simulink model "IntelligentBinPicking"  (R2023a)
settings: Solver=FixedStepAuto  StartTime=0.0  StopTime=100  FixedStep=0.1  RelTol=1e-3
PreLoadFcn:
  | initializeParametersForBinPickingSimulationSL;
model workspace (MAT data in the model file):
  SL_ROS_VariableLengthArrays_MaxSizes.CommonInfo.ArrayTruncateAction = 'EmitWarning'
  SL_ROS_VariableLengthArrays_MaxSizes.MsgTypeMap = containers.Map
  SL_ROS_VariableLengthArrays_MaxSizes.MsgTypeMap.serialization.keys = {'sensor_msgs/Image', 'sensor_msgs/PointCloud2'}
  SL_ROS_VariableLengthArrays_MaxSizes.MsgTypeMap.serialization.values{1}(1).PropertyName = 'Data'
  SL_ROS_VariableLengthArrays_MaxSizes.MsgTypeMap.serialization.values{1}(1).DataType = 'uint8'
  SL_ROS_VariableLengthArrays_MaxSizes.MsgTypeMap.serialization.values{1}(1).MaxLength = 921600
  SL_ROS_VariableLengthArrays_MaxSizes.MsgTypeMap.serialization.values{1}(2).PropertyName = 'Encoding'
  SL_ROS_VariableLengthArrays_MaxSizes.MsgTypeMap.serialization.values{1}(2).DataType = 'uint8'
  SL_ROS_VariableLengthArrays_MaxSizes.MsgTypeMap.serialization.values{1}(2).MaxLength = 128
  SL_ROS_VariableLengthArrays_MaxSizes.MsgTypeMap.serialization.values{2}(1).PropertyName = 'Data'
  SL_ROS_VariableLengthArrays_MaxSizes.MsgTypeMap.serialization.values{2}(1).DataType = 'uint8'
  SL_ROS_VariableLengthArrays_MaxSizes.MsgTypeMap.serialization.values{2}(1).MaxLength = 9830400
  SL_ROS_VariableLengthArrays_MaxSizes.MsgTypeMap.serialization.values{2}(2).PropertyName = 'Fields'
  SL_ROS_VariableLengthArrays_MaxSizes.MsgTypeMap.serialization.values{2}(2).DataType = 'sensor_msgs/PointField'
  SL_ROS_VariableLengthArrays_MaxSizes.MsgTypeMap.serialization.values{2}(2).MaxLength = 16
  SL_ROS_VariableLengthArrays_MaxSizes.MsgTypeMap.serialization.uniformity = 0
  SL_ROS_VariableLengthArrays_MaxSizes.MsgTypeMap.serialization.keyType = 'char'
  SL_ROS_VariableLengthArrays_MaxSizes.MsgTypeMap.serialization.valueType = 'any'
undefined symbols (not defined in the file): binCenterPosition, Enable, enumCmd, homePosition, IsAccValid, IsMoving, IsPosValid, isSingleDetection, IsValid, IsVelValid, JointAcc, JointCurrent, JointPos, JointTrajectory, JointVel, maxVisionObjects, Mode, motionPlannerCmdInitValue, motionPlannerResponseInitValue, NumObjects, NumPoints, objectDetectorResponseInitValue, Objects, ObjectTypesID, PickAllOrder, pickAllOrder, PickAndPlaceModes, PickSelectedObjectID, posTargetError, RequestID, Reset, RGBCameraTransform, robotCommandInitValue, robotFeedbackInitValue, Status, targetEnv, TaskPlannerSampleTime, Time, TooltipTransform
libraries: robotlib x10, robotmaniplib x3, visionanalysis x2, robotcorelib x1, visiontextngfix x1, visionsinks x1
(part 1 of 2)
settings Model: Creator=gjohn  LastModifiedBy=amathamk
settings DebuggingCC: SubsystemReferenceDiagnosticForUnitTest=warning

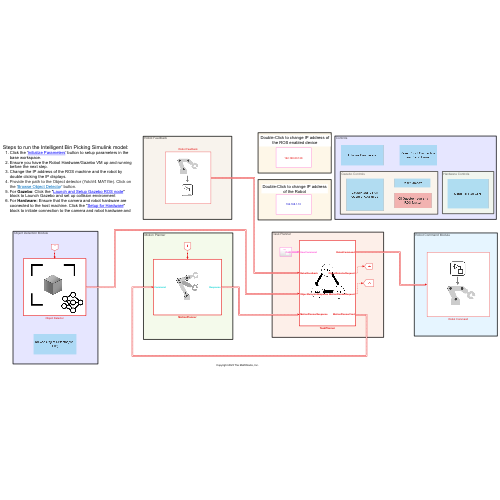
[thumbnail: Simulink's stored preview of the top-level diagram]
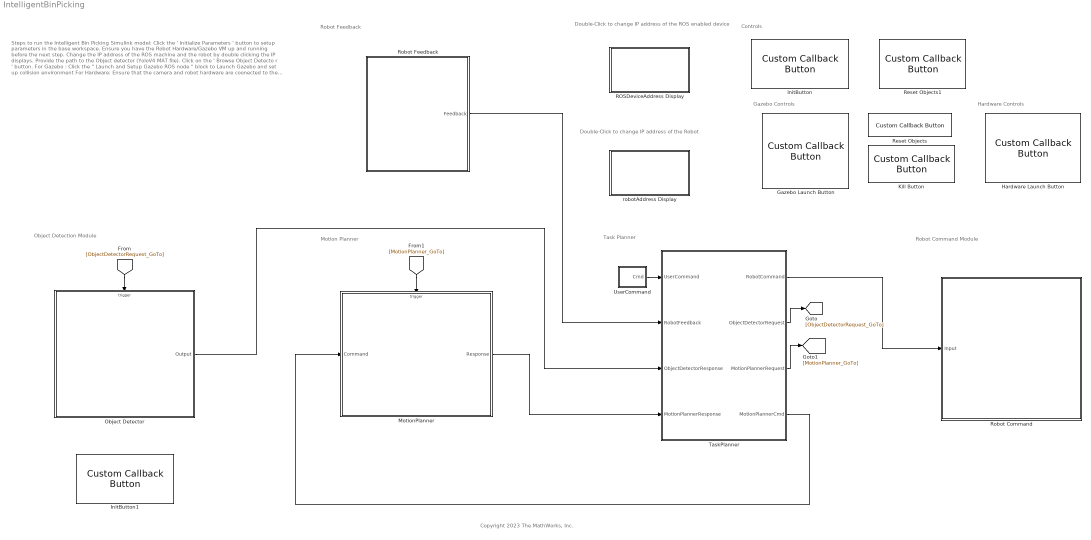
== system IntelligentBinPicking ==
  note: Double-Click to change IP address of the ROS enabled device
  note: Gazebo Controls
  note: Steps to run the Intelligent Bin Picking Simulink model:
      | Click the ' Initialize Parameters ' button to setup parameters in the base workspace.
      | Ensure you have the Robot Hardware/Gazebo VM up and running before the next step.
      | Change the IP address of the ROS machine and the robot by double clicking the IP displays.
      | Provide the path to the Object detector (YoloV4 MAT file). Click on the ' Browse Object Detecto r ' button.
      | For Gazebo : Click the " Launch and Setup Gazebo ROS node " block to Launch Gazebo and set up collision environment
      | For Hardware: Ensure that the camera and robot hardware are coonected to the host machine. Click the " Setup for Hardware " block to initiate connection to the camera and robot hardware and call rosinit.
  note: Task Planner
  note: Motion Planner
  note: Robot Command Module
  note: Robot Feedback
  note: Object Detection Module
  note: Controls
  note: Copyright 2023 The MathWorks, Inc.
  note: Hardware Controls
  note: Double-Click to change IP address of the Robot
  Gazebo Launch Button : CustomCallbackButton  Configuration="{\"components\":[{\"name\":\"BackgroundImageComponent\",\"settings\":{\"image\":{\"size\":[0,0],\"src\":\"default\",\"srcOrientation\":\"Right\"},\"position\":[0,0,1,1]}},{\"name\":\"ButtonStateComponent\",\"settings\":{\"buttonType\":\"momentary\",\"clickFcn\":\"LaunchGazeboAndSetupCollisionEnv;\\ndisp(\\\"Gazebo launched and scene setup\\\")\\n\",\"onValue\":1,\"position\":[0,0,1,1],\"pressDelay\":\"500\",\"pressFcn\":\"\",\"repeatInterval\":\"0\",\"states\":[{\"horizontalAlignment\":\"center\",\"image\":{\"position\":[0,0,1,1],\"size\":[1,1],\"src\":\"default\",\"srcOrientation\":\"Right\"},\"label\":{\"color\":[0.01176470588,0.01176470588,0.01176470588,1],\"icon\":{\"size\":[0,0],\"src\":\"default\",\"srcOrientation\":\"Right\"},\"iconPlacement\":\"left\",\"opacity\":1,\"show\":true,\"text\":{\"content\":\"Launch and Setup Gazebo ROS node\",\"font\":\"Helvetica\",\"fontSize\":9.600000000000001}},\"labelOffset\":[0,0],\"verticalAlignment\":\"middle\"},{\"horizontalAlignment\":\"center\",\"image\":{\"position\":[0,0,1,1],\"size\":[1,1],\"src\":\"default\",\"srcOrientation\":\"Right\"},\"label\":{\"color\":[0.01176470588,0.01176470588,0.01176470588,1],\"icon\":{\"size\":[0,0],\"src\":\"default\",\"srcOrientation\":\"Right\"},\"iconPlacement\":\"left\",\"opacity\":1,\"show\":true,\"text\":{\"content\":\"Launch and Setup Gazebo ROS node\",\"font\":\"Helvetica\",\"fontSize\":9.600000000000001}},\"labelOffset\":[0,0],\"verticalAlignment\":\"middle\"},{\"horizontalAlignment\":\"center\",\"image\":{\"position\":[0,0,1,1],\"size\":[1,1],\"src\":\"default\",\"srcOrientation\":\"Right\"},\"label\":{\"color\":[0.01176470588,0.01176470588,0.01176470588,1],\"icon\":{\"size\":[0,0],\"src\":\"default\",\"srcOrientation\":\"Right\"},\"iconPlacement\":\"left\",\"opacity\":1,\"show\":true,\"text\":{\"content\":\"Launch and Setup Gazebo ROS node\",\"font\":\"Helvetica\",\"fontSize\":9.600000000000001}},\"labelOffset\":[0,0],\"verticalAlignment\":\"middle\"},{\"horizontalAlignment\":\"center\",\"image\":{\"position\":[0,0,1,1],\"size\":[1,1],\"src\":\"default\",\"srcOrientation\":\"Right\"},\"label\":{\"color\":[0.01176470588,0.01176470588,0.01176470588,1],\"icon\":{\"size\":[0,0],\"src\":\"default\",\"srcOrientation\":\"Right\"},\"iconPlacement\":\"left\",\"opacity\":1,\"show\":true,\"text\":{\"content\":\"Launch and Setup Gazebo ROS node\",\"font\":\"Helvetica\",\"fontSize\":9.600000000000001}},\"labelOffset\":[0,0],\"verticalAlignment\":\"middle\"}]}},{\"name\":\"ForegroundImageComponent\",\"settings\":{\"image\":{\"size\":[0,0],\"src\":\"default\",\"srcOrientation\":\"Right\"},\"isForeground\":1,\"position\":[0,0,1,1]}}],\"settings\":{\"BindingType\":\"standalone\",\"backgroundColor\":[244,244,244,1],\"backgroundOffset\":0,\"backgroundOpacity\":1,\"fixedAspectRatio\":\"off\",\"foregroundColor\":[0.01176470588,0.01176470588,0.01176470588,1],\"migratedFromLegacy\":true,\"useBackgroundColor\":true,\"variant\":\"callback\",\"version\":\"R2023a\"},\"type\":\"Button\"}"  CustomBackgroundColor="{\"color\":[0.6196078431372549,0.8392156862745098,0.9490196078431372],\"show\":true}"
  Hardware Launch Button : CustomCallbackButton  Configuration="{\"components\":[{\"name\":\"BackgroundImageComponent\",\"settings\":{\"image\":{\"size\":[0,0],\"src\":\"default\",\"srcOrientation\":\"Right\"},\"position\":[0,0,1,1]}},{\"name\":\"ButtonStateComponent\",\"settings\":{\"buttonType\":\"momentary\",\"clickFcn\":\"getGripperType;\\n\\nConnectToRobotROS;\\n\\ndisp(\\\"Setup complete for Robot hardware\\\")\\n\",\"onValue\":1,\"position\":[0,0,1,1],\"pressDelay\":\"500\",\"pressFcn\":\"\",\"repeatInterval\":\"0\",\"states\":[{\"horizontalAlignment\":\"center\",\"image\":{\"position\":[0,0,1,1],\"size\":[1,1],\"src\":\"default\",\"srcOrientation\":\"Right\"},\"label\":{\"color\":[0.011764705882352941,0.011764705882352941,0.011764705882352941],\"icon\":{\"size\":[0,0],\"src\":\"default\",\"srcOrientation\":\"Right\"},\"iconPlacement\":\"left\",\"opacity\":1,\"show\":true,\"text\":{\"content\":\"Setup for Hardware\",\"font\":\"Helvetica\",\"fontSize\":11.709468000000001}},\"labelOffset\":[0,0],\"verticalAlignment\":\"middle\"},{\"horizontalAlignment\":\"center\",\"image\":{\"position\":[0,0,1,1],\"size\":[1,1],\"src\":\"default\",\"srcOrientation\":\"Right\"},\"label\":{\"color\":[0.011764705882352941,0.011764705882352941,0.011764705882352941],\"icon\":{\"size\":[0,0],\"src\":\"default\",\"srcOrientation\":\"Right\"},\"iconPlacement\":\"left\",\"opacity\":1,\"show\":true,\"text\":{\"content\":\"Setup for Hardware\",\"font\":\"Helvetica\",\"fontSize\":11.709468000000001}},\"labelOffset\":[0,0],\"verticalAlignment\":\"middle\"},{\"horizontalAlignment\":\"center\",\"image\":{\"position\":[0,0,1,1],\"size\":[1,1],\"src\":\"default\",\"srcOrientation\":\"Right\"},\"label\":{\"color\":[0.011764705882352941,0.011764705882352941,0.011764705882352941],\"icon\":{\"size\":[0,0],\"src\":\"default\",\"srcOrientation\":\"Right\"},\"iconPlacement\":\"left\",\"opacity\":1,\"show\":true,\"text\":{\"content\":\"Setup for Hardware\",\"font\":\"Helvetica\",\"fontSize\":11.709468000000001}},\"labelOffset\":[0,0],\"verticalAlignment\":\"middle\"},{\"horizontalAlignment\":\"center\",\"image\":{\"position\":[0,0,1,1],\"size\":[1,1],\"src\":\"default\",\"srcOrientation\":\"Right\"},\"label\":{\"color\":[0.011764705882352941,0.011764705882352941,0.011764705882352941],\"icon\":{\"size\":[0,0],\"src\":\"default\",\"srcOrientation\":\"Right\"},\"iconPlacement\":\"left\",\"opacity\":1,\"show\":true,\"text\":{\"content\":\"Setup for Hardware\",\"font\":\"Helvetica\",\"fontSize\":11.709468000000001}},\"labelOffset\":[0,0],\"verticalAlignment\":\"middle\"}]}},{\"name\":\"ForegroundImageComponent\",\"settings\":{\"image\":{\"size\":[0,0],\"src\":\"default\",\"srcOrientation\":\"Right\"},\"isForeground\":1,\"position\":[0,0,1,1]}}],\"settings\":{\"BindingType\":\"standalone\",\"backgroundColor\":[244,244,244,1],\"backgroundOffset\":0,\"backgroundOpacity\":1,\"fixedAspectRatio\":\"off\",\"foregroundColor\":[0.01176470588,0.01176470588,0.01176470588,1],\"migratedFromLegacy\":true,\"useBackgroundColor\":true,\"variant\":\"callback\",\"version\":\"R2023a\"},\"type\":\"Button\"}"  CustomBackgroundColor="{\"color\":[0.6196078431372549,0.8392156862745098,0.9490196078431372],\"show\":true}"
  InitButton : CustomCallbackButton  Configuration="{\"components\":[{\"name\":\"BackgroundImageComponent\",\"settings\":{\"image\":{\"size\":[0,0],\"src\":\"default\",\"srcOrientation\":\"Right\"},\"position\":[0,0,1,1]}},{\"name\":\"ButtonStateComponent\",\"settings\":{\"buttonType\":\"momentary\",\"clickFcn\":\"%%\\ninitializeParametersForBinPickingSimulationSL;\\ndisp('Parameters Initialized')\",\"onValue\":1,\"position\":[0,0,1,1],\"pressDelay\":\"500\",\"pressFcn\":\"\",\"repeatInterval\":\"0\",\"states\":[{\"horizontalAlignment\":\"center\",\"image\":{\"position\":[0,0,1,1],\"size\":[1,1],\"src\":\"default\",\"srcOrientation\":\"Right\"},\"label\":{\"color\":[0,0,0],\"icon\":{\"size\":[0,0],\"src\":\"default\",\"srcOrientation\":\"Right\"},\"iconPlacement\":\"left\",\"opacity\":1,\"show\":true,\"text\":{\"content\":\"Initialize Parameters\",\"font\":\"Helvetica\",\"fontSize\":11.709468000000001}},\"labelOffset\":[0,0],\"verticalAlignment\":\"middle\"},{\"horizontalAlignment\":\"center\",\"image\":{\"position\":[0,0,1,1],\"size\":[1,1],\"src\":\"default\",\"srcOrientation\":\"Right\"},\"label\":{\"color\":[0.01176470588,0.01176470588,0.01176470588,1],\"icon\":{\"size\":[0,0],\"src\":\"default\",\"srcOrientation\":\"Right\"},\"iconPlacement\":\"left\",\"opacity\":1,\"show\":true,\"text\":{\"content\":\"Initialize Parameters\",\"font\":\"Helvetica\",\"fontSize\":11.709468000000001}},\"labelOffset\":[0,0],\"verticalAlignment\":\"middle\"},{\"horizontalAlignment\":\"center\",\"image\":{\"position\":[0,0,1,1],\"size\":[1,1],\"src\":\"default\",\"srcOrientation\":\"Right\"},\"label\":{\"color\":[0.01176470588,0.01176470588,0.01176470588,1],\"icon\":{\"size\":[0,0],\"src\":\"default\",\"srcOrientation\":\"Right\"},\"iconPlacement\":\"left\",\"opacity\":1,\"show\":true,\"text\":{\"content\":\"Initialize Parameters\",\"font\":\"Helvetica\",\"fontSize\":11.709468000000001}},\"labelOffset\":[0,0],\"verticalAlignment\":\"middle\"},{\"horizontalAlignment\":\"center\",\"image\":{\"position\":[0,0,1,1],\"size\":[1,1],\"src\":\"default\",\"srcOrientation\":\"Right\"},\"label\":{\"color\":[0.01176470588,0.01176470588,0.01176470588,1],\"icon\":{\"size\":[0,0],\"src\":\"default\",\"srcOrientation\":\"Right\"},\"iconPlacement\":\"left\",\"opacity\":1,\"show\":true,\"text\":{\"content\":\"Initialize Parameters\",\"font\":\"Helvetica\",\"fontSize\":11.709468000000001}},\"labelOffset\":[0,0],\"verticalAlignment\":\"middle\"}]}},{\"name\":\"ForegroundImageComponent\",\"settings\":{\"image\":{\"size\":[0,0],\"src\":\"default\",\"srcOrientation\":\"Right\"},\"isForeground\":1,\"position\":[0,0,1,1]}}],\"settings\":{\"BindingType\":\"standalone\",\"backgroundColor\":[244,244,244,1],\"backgroundOffset\":0,\"backgroundOpacity\":1,\"fixedAspectRatio\":\"off\",\"foregroundColor\":[0.01176470588,0.01176470588,0.01176470588,1],\"migratedFromLegacy\":true,\"useBackgroundColor\":true,\"variant\":\"callback\",\"version\":\"R2023a\"},\"type\":\"Button\"}"  CustomBackgroundColor="{\"color\":[0.6196078431372549,0.8392156862745098,0.9490196078431372],\"show\":true}"
  InitButton1 : CustomCallbackButton  Configuration="{\"components\":[{\"name\":\"BackgroundImageComponent\",\"settings\":{\"image\":{\"size\":[0,0],\"src\":\"default\",\"srcOrientation\":\"Right\"},\"position\":[0,0,1,1]}},{\"name\":\"ButtonStateComponent\",\"settings\":{\"buttonType\":\"momentary\",\"clickFcn\":\"selectDetectorMATFile\",\"onValue\":1,\"position\":[0,0,1,1],\"pressDelay\":\"500\",\"pressFcn\":\"\",\"repeatInterval\":\"0\",\"states\":[{\"horizontalAlignment\":\"center\",\"image\":{\"position\":[0,0,1,1],\"size\":[1,1],\"src\":\"default\",\"srcOrientation\":\"Right\"},\"label\":{\"color\":[0,0,0],\"icon\":{\"size\":[0,0],\"src\":\"default\",\"srcOrientation\":\"Right\"},\"iconPlacement\":\"left\",\"opacity\":1,\"show\":true,\"text\":{\"content\":\"Browse Object Detector(MAT File)\",\"font\":\"Helvetica\",\"fontSize\":10.608108000000001}},\"labelOffset\":[0,0],\"verticalAlignment\":\"middle\"},{\"horizontalAlignment\":\"center\",\"image\":{\"position\":[0,0,1,1],\"size\":[1,1],\"src\":\"default\",\"srcOrientation\":\"Right\"},\"label\":{\"color\":[0.01176470588,0.01176470588,0.01176470588,1],\"icon\":{\"size\":[0,0],\"src\":\"default\",\"srcOrientation\":\"Right\"},\"iconPlacement\":\"left\",\"opacity\":1,\"show\":true,\"text\":{\"content\":\"Browse Object Detector(MAT File)\",\"font\":\"Helvetica\",\"fontSize\":10.608108000000001}},\"labelOffset\":[0,0],\"verticalAlignment\":\"middle\"},{\"horizontalAlignment\":\"center\",\"image\":{\"position\":[0,0,1,1],\"size\":[1,1],\"src\":\"default\",\"srcOrientation\":\"Right\"},\"label\":{\"color\":[0.01176470588,0.01176470588,0.01176470588,1],\"icon\":{\"size\":[0,0],\"src\":\"default\",\"srcOrientation\":\"Right\"},\"iconPlacement\":\"left\",\"opacity\":1,\"show\":true,\"text\":{\"content\":\"Browse Object Detector(MAT File)\",\"font\":\"Helvetica\",\"fontSize\":10.608108000000001}},\"labelOffset\":[0,0],\"verticalAlignment\":\"middle\"},{\"horizontalAlignment\":\"center\",\"image\":{\"position\":[0,0,1,1],\"size\":[1,1],\"src\":\"default\",\"srcOrientation\":\"Right\"},\"label\":{\"color\":[0.01176470588,0.01176470588,0.01176470588,1],\"icon\":{\"size\":[0,0],\"src\":\"default\",\"srcOrientation\":\"Right\"},\"iconPlacement\":\"left\",\"opacity\":1,\"show\":true,\"text\":{\"content\":\"Browse Object Detector(MAT File)\",\"font\":\"Helvetica\",\"fontSize\":10.608108000000001}},\"labelOffset\":[0,0],\"verticalAlignment\":\"middle\"}]}},{\"name\":\"ForegroundImageComponent\",\"settings\":{\"image\":{\"size\":[0,0],\"src\":\"default\",\"srcOrientation\":\"Right\"},\"isForeground\":1,\"position\":[0,0,1,1]}}],\"settings\":{\"BindingType\":\"standalone\",\"backgroundColor\":[244,244,244,1],\"backgroundOffset\":0,\"backgroundOpacity\":1,\"fixedAspectRatio\":\"off\",\"foregroundColor\":[0.01176470588,0.01176470588,0.01176470588,1],\"migratedFromLegacy\":true,\"useBackgroundColor\":true,\"variant\":\"callback\",\"version\":\"R2023a\"},\"type\":\"Button\"}"  CustomBackgroundColor="{\"color\":[0.6196078431372549,0.8392156862745098,0.9490196078431372],\"show\":true}"
  Kill Button : CustomCallbackButton  Configuration="{\"components\":[{\"name\":\"BackgroundImageComponent\",\"settings\":{\"image\":{\"size\":[0,0],\"src\":\"default\",\"srcOrientation\":\"Right\"},\"position\":[0,0,1,1]}},{\"name\":\"ButtonStateComponent\",\"settings\":{\"buttonType\":\"momentary\",\"clickFcn\":\"clear ur\\nurHandleClass.manageURNodeMap(ROSDeviceAddress,[],'remove')\\nif exist('device', 'var')\\n    system(device,'killall -9 rosmaster');\\nend\",\"onValue\":1,\"position\":[0,0,1,1],\"pressDelay\":\"500\",\"pressFcn\":\"\",\"repeatInterval\":\"0\",\"states\":[{\"horizontalAlignment\":\"center\",\"image\":{\"position\":[0,0,1,1],\"size\":[1,1],\"src\":\"default\",\"srcOrientation\":\"Right\"},\"label\":{\"color\":[0,0,0],\"icon\":{\"size\":[0,0],\"src\":\"default\",\"srcOrientation\":\"Right\"},\"iconPlacement\":\"left\",\"opacity\":1,\"show\":true,\"text\":{\"content\":\"Kill Gazebo node and ROS Master\",\"font\":\"Helvetica\",\"fontSize\":14.45202}},\"labelOffset\":[0,0],\"verticalAlignment\":\"middle\"},{\"horizontalAlignment\":\"center\",\"image\":{\"position\":[0,0,1,1],\"size\":[1,1],\"src\":\"default\",\"srcOrientation\":\"Right\"},\"label\":{\"color\":[0.01176470588,0.01176470588,0.01176470588,1],\"icon\":{\"size\":[0,0],\"src\":\"default\",\"srcOrientation\":\"Right\"},\"iconPlacement\":\"left\",\"opacity\":1,\"show\":true,\"text\":{\"content\":\"Kill Gazebo node and ROS Master\",\"font\":\"Helvetica\",\"fontSize\":14.45202}},\"labelOffset\":[0,0],\"verticalAlignment\":\"middle\"},{\"horizontalAlignment\":\"center\",\"image\":{\"position\":[0,0,1,1],\"size\":[1,1],\"src\":\"default\",\"srcOrientation\":\"Right\"},\"label\":{\"color\":[0.01176470588,0.01176470588,0.01176470588,1],\"icon\":{\"size\":[0,0],\"src\":\"default\",\"srcOrientation\":\"Right\"},\"iconPlacement\":\"left\",\"opacity\":1,\"show\":true,\"text\":{\"content\":\"Kill Gazebo node and ROS Master\",\"font\":\"Helvetica\",\"fontSize\":14.45202}},\"labelOffset\":[0,0],\"verticalAlignment\":\"middle\"},{\"horizontalAlignment\":\"center\",\"image\":{\"position\":[0,0,1,1],\"size\":[1,1],\"src\":\"default\",\"srcOrientation\":\"Right\"},\"label\":{\"color\":[0.01176470588,0.01176470588,0.01176470588,1],\"icon\":{\"size\":[0,0],\"src\":\"default\",\"srcOrientation\":\"Right\"},\"iconPlacement\":\"left\",\"opacity\":1,\"show\":true,\"text\":{\"content\":\"Kill Gazebo node and ROS Master\",\"font\":\"Helvetica\",\"fontSize\":14.45202}},\"labelOffset\":[0,0],\"verticalAlignment\":\"middle\"}]}},{\"name\":\"ForegroundImageComponent\",\"settings\":{\"image\":{\"size\":[0,0],\"src\":\"default\",\"srcOrientation\":\"Right\"},\"isForeground\":1,\"position\":[0,0,1,1]}}],\"settings\":{\"BindingType\":\"standalone\",\"backgroundColor\":[244,244,244,1],\"backgroundOffset\":0,\"backgroundOpacity\":1,\"fixedAspectRatio\":\"off\",\"foregroundColor\":[0.01176470588,0.01176470588,0.01176470588,1],\"migratedFromLegacy\":true,\"useBackgroundColor\":true,\"variant\":\"callback\",\"version\":\"R2023a\"},\"type\":\"Button\"}"  CustomBackgroundColor="{\"color\":[0.9411764705882353,0.6313725490196078,0.6313725490196078],\"show\":true}"
  MotionPlanner : Subsystem
      mask Display: image('$imagefile'); % Use "Edit Image" on toolstrip to change.
  Object Detector : Subsystem  TreatAsAtomicUnit=on
      mask Display: image('$imagefile'); % Use "Edit Image" on toolstrip to change.
  ROSDeviceAddress Display : Subsystem
      settings: OpenFcn=RequestIP;
      mask Display: color('red'); try ipad = evalin('base', 'ROSDeviceAddress'); catch ipad = '0.0.0.0'; end; disp(ipad)
  Reset Objects : CustomCallbackButton  Configuration="{\"components\":[{\"name\":\"BackgroundImageComponent\",\"settings\":{\"image\":{\"size\":[0,0],\"src\":\"default\",\"srcOrientation\":\"Right\"},\"position\":[0,0,1,1]}},{\"name\":\"ButtonStateComponent\",\"settings\":{\"buttonType\":\"momentary\",\"clickFcn\":\"ResetObjectsGazebo;\\ndisp(\\\"Object positions and collision environment reset\\\")\",\"onValue\":1,\"position\":[0,0,1,1],\"pressDelay\":\"500\",\"pressFcn\":\"\",\"repeatInterval\":\"0\",\"states\":[{\"horizontalAlignment\":\"center\",\"image\":{\"position\":[0,0,1,1],\"size\":[1,1],\"src\":\"default\",\"srcOrientation\":\"Right\"},\"label\":{\"color\":[0,0,0],\"icon\":{\"size\":[0,0],\"src\":\"default\",\"srcOrientation\":\"Right\"},\"iconPlacement\":\"left\",\"opacity\":1,\"show\":true,\"text\":{\"content\":\"Reset Objects\",\"font\":\"Helvetica\",\"fontSize\":15}},\"labelOffset\":[0,0],\"verticalAlignment\":\"middle\"},{\"horizontalAlignment\":\"center\",\"image\":{\"position\":[0,0,1,1],\"size\":[1,1],\"src\":\"default\",\"srcOrientation\":\"Right\"},\"label\":{\"color\":[0.01176470588,0.01176470588,0.01176470588,1],\"icon\":{\"size\":[0,0],\"src\":\"default\",\"srcOrientation\":\"Right\"},\"iconPlacement\":\"left\",\"opacity\":1,\"show\":true,\"text\":{\"content\":\"Reset Objects\",\"font\":\"Helvetica\",\"fontSize\":15}},\"labelOffset\":[0,0],\"verticalAlignment\":\"middle\"},{\"horizontalAlignment\":\"center\",\"image\":{\"position\":[0,0,1,1],\"size\":[1,1],\"src\":\"default\",\"srcOrientation\":\"Right\"},\"label\":{\"color\":[0.01176470588,0.01176470588,0.01176470588,1],\"icon\":{\"size\":[0,0],\"src\":\"default\",\"srcOrientation\":\"Right\"},\"iconPlacement\":\"left\",\"opacity\":1,\"show\":true,\"text\":{\"content\":\"Reset Objects\",\"font\":\"Helvetica\",\"fontSize\":15}},\"labelOffset\":[0,0],\"verticalAlignment\":\"middle\"},{\"horizontalAlignment\":\"center\",\"image\":{\"position\":[0,0,1,1],\"size\":[1,1],\"src\":\"default\",\"srcOrientation\":\"Right\"},\"label\":{\"color\":[0.01176470588,0.01176470588,0.01176470588,1],\"icon\":{\"size\":[0,0],\"src\":\"default\",\"srcOrientation\":\"Right\"},\"iconPlacement\":\"left\",\"opacity\":1,\"show\":true,\"text\":{\"content\":\"Reset Objects\",\"font\":\"Helvetica\",\"fontSize\":15}},\"labelOffset\":[0,0],\"verticalAlignment\":\"middle\"}]}},{\"name\":\"ForegroundImageComponent\",\"settings\":{\"image\":{\"size\":[0,0],\"src\":\"default\",\"srcOrientation\":\"Right\"},\"isForeground\":1,\"position\":[0,0,1,1]}}],\"settings\":{\"BindingType\":\"standalone\",\"backgroundColor\":[244,244,244,1],\"backgroundOffset\":0,\"backgroundOpacity\":1,\"fixedAspectRatio\":\"off\",\"foregroundColor\":[0.01176470588,0.01176470588,0.01176470588,1],\"migratedFromLegacy\":true,\"useBackgroundColor\":true,\"variant\":\"callback\",\"version\":\"R2023a\"},\"type\":\"Button\"}"  CustomBackgroundColor="{\"color\":[0.6196078431372549,0.8392156862745098,0.9490196078431372],\"show\":true}"
  Reset Objects1 : CustomCallbackButton  Configuration="{\"components\":[{\"name\":\"BackgroundImageComponent\",\"settings\":{\"image\":{\"size\":[0,0],\"src\":\"default\",\"srcOrientation\":\"Right\"},\"position\":[0,0,1,1]}},{\"name\":\"ButtonStateComponent\",\"settings\":{\"buttonType\":\"momentary\",\"clickFcn\":\"urHandleClass.manageURNodeMap(ROSDeviceAddress,[],'remove');\\nif exist('ur', 'var')\\n    clear ur\\nend\\nur = universalrobot(ROSDeviceAddress,'RigidBodyTree',ur5e);\\nsendJointConfigurationAndWait(ur,homePosition,'EndTime',2);\\npause(2);\\nclear ur\\ndisp(\\\"Robot connection reset\\\")\",\"onValue\":1,\"position\":[0,0,1,1],\"pressDelay\":\"500\",\"pressFcn\":\"\",\"repeatInterval\":\"0\",\"states\":[{\"horizontalAlignment\":\"center\",\"image\":{\"position\":[0,0,1,1],\"size\":[1,1],\"src\":\"default\",\"srcOrientation\":\"Right\"},\"label\":{\"color\":[0,0,0],\"icon\":{\"size\":[0,0],\"src\":\"default\",\"srcOrientation\":\"Right\"},\"iconPlacement\":\"left\",\"opacity\":1,\"show\":true,\"text\":{\"content\":\"Reset Robot Connection and Send Home\",\"font\":\"Helvetica\",\"fontSize\":14.45202}},\"labelOffset\":[0,0],\"verticalAlignment\":\"middle\"},{\"horizontalAlignment\":\"center\",\"image\":{\"position\":[0,0,1,1],\"size\":[1,1],\"src\":\"default\",\"srcOrientation\":\"Right\"},\"label\":{\"color\":[0.01176470588,0.01176470588,0.01176470588,1],\"icon\":{\"size\":[0,0],\"src\":\"default\",\"srcOrientation\":\"Right\"},\"iconPlacement\":\"left\",\"opacity\":1,\"show\":true,\"text\":{\"content\":\"Reset Robot Connection and Send Home\",\"font\":\"Helvetica\",\"fontSize\":14.45202}},\"labelOffset\":[0,0],\"verticalAlignment\":\"middle\"},{\"horizontalAlignment\":\"center\",\"image\":{\"position\":[0,0,1,1],\"size\":[1,1],\"src\":\"default\",\"srcOrientation\":\"Right\"},\"label\":{\"color\":[0.01176470588,0.01176470588,0.01176470588,1],\"icon\":{\"size\":[0,0],\"src\":\"default\",\"srcOrientation\":\"Right\"},\"iconPlacement\":\"left\",\"opacity\":1,\"show\":true,\"text\":{\"content\":\"Reset Robot Connection and Send Home\",\"font\":\"Helvetica\",\"fontSize\":14.45202}},\"labelOffset\":[0,0],\"verticalAlignment\":\"middle\"},{\"horizontalAlignment\":\"center\",\"image\":{\"position\":[0,0,1,1],\"size\":[1,1],\"src\":\"default\",\"srcOrientation\":\"Right\"},\"label\":{\"color\":[0.01176470588,0.01176470588,0.01176470588,1],\"icon\":{\"size\":[0,0],\"src\":\"default\",\"srcOrientation\":\"Right\"},\"iconPlacement\":\"left\",\"opacity\":1,\"show\":true,\"text\":{\"content\":\"Reset Robot Connection and Send Home\",\"font\":\"Helvetica\",\"fontSize\":14.45202}},\"labelOffset\":[0,0],\"verticalAlignment\":\"middle\"}]}},{\"name\":\"ForegroundImageComponent\",\"settings\":{\"image\":{\"size\":[0,0],\"src\":\"default\",\"srcOrientation\":\"Right\"},\"isForeground\":1,\"position\":[0,0,1,1]}}],\"settings\":{\"BindingType\":\"standalone\",\"backgroundColor\":[244,244,244,1],\"backgroundOffset\":0,\"backgroundOpacity\":1,\"fixedAspectRatio\":\"off\",\"foregroundColor\":[0.01176470588,0.01176470588,0.01176470588,1],\"migratedFromLegacy\":true,\"useBackgroundColor\":true,\"variant\":\"callback\",\"version\":\"R2023a\"},\"type\":\"Button\"}"  CustomBackgroundColor="{\"color\":[0.615686274509804,0.8392156862745098,0.9490196078431372],\"show\":true}"
  Robot Command : Subsystem
      mask Display: image('SLToRobotComm.png'); % Use "Edit Image" on toolstrip to change.
  Robot Feedback : Subsystem
      mask Display: image('$imagefile'); % Use "Edit Image" on toolstrip to change.
  TaskPlanner : Subsystem  TreatAsAtomicUnit=on  SystemSampleTime=TaskPlannerSampleTime
      mask Display: image('$imagefile'); % Use "Edit Image" on toolstrip to change.
  UserCommand : Subsystem
  robotAddress Display : Subsystem
      settings: OpenFcn=RequestRobotIP;
      mask Display: color('blue'); try ipad = evalin('base', 'robotAddress'); catch ipad = '192.162.1.10'; end; disp(ipad)
  wires:
  UserCommand/1(Cmd) -> TaskPlanner/1(UserCommand)
  TaskPlanner/2(ObjectDetectorRequest) -> [ObjectDetectorRequest_GoTo]
  [ObjectDetectorRequest_GoTo] -> Object Detector/Trigger
  TaskPlanner/3(MotionPlannerRequest) -> [MotionPlanner_GoTo]
  [MotionPlanner_GoTo] -> MotionPlanner/Trigger
  TaskPlanner/1(RobotCommand) -> Robot Command/1(Input)
  TaskPlanner/4(MotionPlannerCmd) -> MotionPlanner/1(Command)
  MotionPlanner/1(Response) -> TaskPlanner/4(MotionPlannerResponse)
  Object Detector/1(Output) -> TaskPlanner/3(ObjectDetectorResponse)
  Robot Feedback/1(Feedback) -> TaskPlanner/2(RobotFeedback)

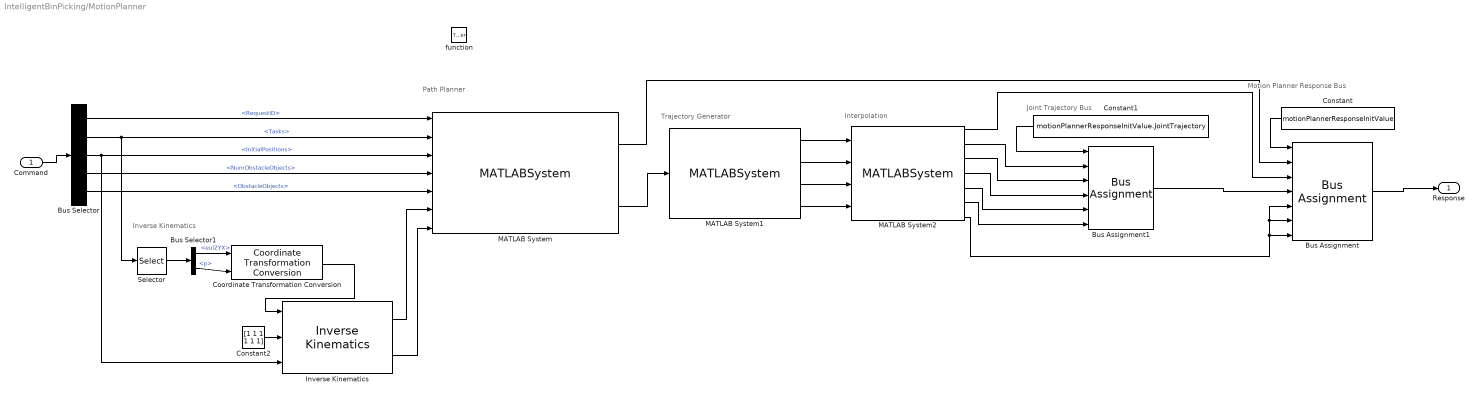
== system IntelligentBinPicking/MotionPlanner ==
  note: Interpolation
  note: Trajectory Generator
  note: Path Planner
  note: Inverse Kinematics
  note: Joint Trajectory Bus
  note: Motion Planner Response Bus
  Command : Inport  OutDataTypeStr=Bus: BUS_motion_planner_cmd
  function : TriggerPort  TriggerType=function-call  VariantControl=Variant  PortDimensions=1
  Bus Assignment : BusAssignment  AssignedSignals=RequestID,Status,JointTrajectory,IsPosValid,IsVelValid,IsAccValid
  Bus Assignment1 : BusAssignment  AssignedSignals=NumPoints,Time,JointPos,JointVel,JointAcc
  Bus Selector : BusSelector  OutputSignals=RequestID,Tasks,InitialPositions,NumObstacleObjects,ObstacleObjects
  Bus Selector1 : BusSelector  OutputSignals=eulZYX,p
  Constant : Constant  Value=motionPlannerResponseInitValue  OutDataTypeStr=Bus: BUS_motion_planner_response
  Constant1 : Constant  Value=motionPlannerResponseInitValue.JointTrajectory  OutDataTypeStr=Bus: BUS_joint_trajectory
  Constant2 : Constant  Value=[1 1 1 1 1 1]
  Coordinate Transformation Conversion : robotcorelib/Coordinate Transformation Conversion  InputRepresentation=Euler Angles  InputEulerSequence=ZYX  ShowTrVecInputPort=on  OutputRepresentation=Homogeneous Transformation  OutputEulerSequence=ZYX  ShowTrVecOutputPort=on  SimulateUsing=Code generation
  Inverse Kinematics : robotmaniplib/Inverse Kinematics  RigidBodyTree=ur5e  EndEffector=tcp  ShowInfo=on  SolverName=BFGS Gradient Projection  EnforceJointLimits=on  MaxIterations=1500  MaxTime=10  GradientTolerance=1e-7  SolutionTolerance=1e-6  StepTolerance=1e-14  ErrorChangeTolerance=1e-12  UseErrorDamping=on  DampingBias=0.0025  SimulateUsing=Code generation
  MATLAB System : MATLABSystem  System=MotionPlannerCHOMPSO  BinLength=binLength  BinHeight=binHeight  BinWidth=binWidth  BinRotation=binRotation  BinCenterPosition=binCenterPosition  HomePosition=retractHomePosition  Target=targetEnv  GripperType=gripperType  IsMEXed=off  SimulateUsing=Interpreted execution
      mask Type: MotionPlannerCHOMPSO
      mask Display:
      | disp('MotionPlannerCHOMPSO');
      | port_label('input',1,'requestID');
      | port_label('input',2,'tasks');
      | port_label('input',3,'q0');
      | port_label('input',4,'numObstacles');
      | port_label('input',5,'obstacles');
      | port_label('input',6,'configSoln');
      | port_label('input',7,'configSolnInfo');
      | port_label('output',1,'reqID');
      | port_label('output',2,'path');
  MATLAB System1 : MATLABSystem  System=ContopptrajSO  VelocityLimits=vellimits  AccelLimits=accellimits  NumSamples=50  SimulateUsing=Code generation
      mask Type: ContopptrajSO
      mask Display:
      | disp('ContopptrajSO');
      | port_label('input',1,'planPath');
      | port_label('output',1,'q');
      | port_label('output',2,'qd');
      | port_label('output',3,'qdd');
      | port_label('output',4,'t');
  MATLAB System2 : MATLABSystem  System=InterpSO  trajectorySampleTime=1/400  MaxNumPoints=maxNumPoints  SimulateUsing=Code generation
      mask Type: InterpSO
      mask Display:
      | disp('InterpSO');
      | port_label('input',1,'q');
      | port_label('input',2,'qd');
      | port_label('input',3,'qdd');
      | port_label('input',4,'t');
      | port_label('output',1,'status');
      | port_label('output',2,'numPoints');
      | port_label('output',3,'time');
      | port_label('output',4,'jointPos');
      | port_label('output',5,'jointVel');
      | port_label('output',6,'jointAcc');
      | port_label('output',7,'isValid');
  Selector : Selector  InputPortWidth=20  IndexOptions=Index vector (dialog)  Indices=1  OutputSizes=1
  Response : Outport  OutDataTypeStr=Bus: BUS_motion_planner_response  InitialOutput=motionPlannerResponseInitValue  VectorParamsAs1DForOutWhenUnconnected=off
  wires:
  Bus Selector1/2 -> Coordinate Transformation Conversion/2  "<p>"
  Bus Selector/3 -> Inverse Kinematics/3, MATLAB System/3  "<InitialPositions>"
  Constant2/1 -> Inverse Kinematics/2
  Selector/1 -> Bus Selector1/1
  Bus Selector/2 -> MATLAB System/2, Selector/1  "<Tasks>"
  Coordinate Transformation Conversion/1 -> Inverse Kinematics/1
  Inverse Kinematics/1 -> MATLAB System/6
  Bus Selector1/1 -> Coordinate Transformation Conversion/1  "<eulZYX>"
  Command/1 -> Bus Selector/1
  Bus Selector/1 -> MATLAB System/1  "<RequestID>"
  MATLAB System2/1 -> Bus Assignment/3
  MATLAB System/1 -> Bus Assignment/2
  MATLAB System2/3 -> Bus Assignment1/3
  MATLAB System2/5 -> Bus Assignment1/5
  MATLAB System2/6 -> Bus Assignment1/6
  Bus Assignment/1 -> Response/1
  Constant1/1 -> Bus Assignment1/1
  MATLAB System2/4 -> Bus Assignment1/4
  MATLAB System2/2 -> Bus Assignment1/2
  Constant/1 -> Bus Assignment/1
  Bus Assignment1/1 -> Bus Assignment/4
  MATLAB System2/7 -> Bus Assignment/5, Bus Assignment/6, Bus Assignment/7
  Bus Selector/4 -> MATLAB System/4  "<NumObstacleObjects>"
  Bus Selector/5 -> MATLAB System/5  "<ObstacleObjects>"
  MATLAB System1/1 -> MATLAB System2/1
  MATLAB System1/2 -> MATLAB System2/2
  MATLAB System1/3 -> MATLAB System2/3
  MATLAB System1/4 -> MATLAB System2/4
  MATLAB System/2 -> MATLAB System1/1
  Inverse Kinematics/2 -> MATLAB System/7

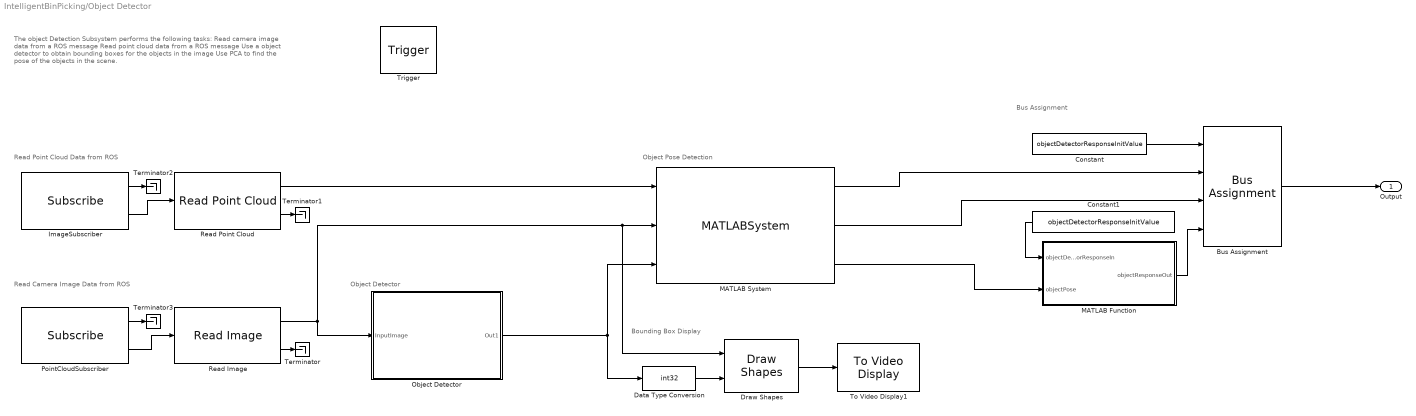
== system IntelligentBinPicking/Object Detector ==
  note: Bounding Box Display
  note: Bus Assignment
  note: The object Detection Subsystem performs the following tasks:
      | Read camera image data from a ROS message
      | Read point cloud data from a ROS message
      | Use a object detector to obtain bounding boxes for the objects in the image
      | Use PCA to find the pose of the objects in the scene.
  note: Object Pose Detection
  note: Read Camera Image Data from ROS
  note: Read Point Cloud Data from ROS
  note: Object Detector
  Trigger : TriggerPort  TriggerType=function-call  VariantControl=(inherit)
  Bus Assignment : BusAssignment  AssignedSignals=Status,NumObjects,Objects
  Constant : Constant  Value=objectDetectorResponseInitValue  OutDataTypeStr=Bus: BUS_object_detector_response
  Constant1 : Constant  Value=objectDetectorResponseInitValue  OutDataTypeStr=Bus: BUS_object_detector_response
  Data Type Conversion : DataTypeConversion  OutDataTypeStr=int32  SaturateOnIntegerOverflow=off  RndMeth=Floor
  Draw Shapes : visiontextngfix/Draw Shapes  shape=Rectangles  fill=off  lineWidth=1  fillClrSource=Specify via dialog  display=Black  intensity=200  color=[200 255 100]  opacity=0.6  viewport=Entire image  antialiasing=off  inType=Obsolete  imagePorts=One multidimensional signal  roundingMode=Floor  overflowMode=off  memoryMode=Specify word length  memoryWordLength=16  prodOutputMode=Binary point scaling  prodOutputWordLength=32  prodOutputFracLength=14  memoryFracLength=15
  ImageSubscriber : robotlib/Subscribe  topicSource=Select from ROS network  topic=/camera/depth/color/points  messageType=sensor_msgs/PointCloud2  SampleTime=-1  legacyBusStruct=off  messageQueueLength=1
  MATLAB Function : MATLAB Function  TreatAsAtomicUnit=on
  MATLAB System : MATLABSystem  System=PerceptionAndLocalizationSO  PlaneThickness=PlaneThickness  normalvector=normalvector  maxPlaneTilt=maxPlaneTilt  gridDownsample=gridDownsample  posDepthCam=posDepthCam  rotationFromRobotToCam=rotationFromRobotToCam  maxVisionObjects=maxVisionObjects  SimulateUsing=Interpreted execution
      mask Type: PerceptionAndLocalizationSO
      mask Display:
      | disp('PerceptionAndLocalizationSO');
      | port_label('input',1,'ptCloudXYZ');
      | port_label('input',2,'rgbImage');
      | port_label('input',3,'bboxes');
      | port_label('output',1,'status');
      | port_label('output',2,'numObjects');
      | port_label('output',3,'objectPose');
  Object Detector : Subsystem  Variant=on
  PointCloudSubscriber : robotlib/Subscribe  topicSource=Select from ROS network  topic=/camera/color/image_raw  messageType=sensor_msgs/Image  SampleTime=-1  legacyBusStruct=off  messageQueueLength=1
  Read Image : robotlib/Read Image  MaximumImageSize=[ 480, 640 ]  ImageEncoding=rgb8  ShowAlphaOutput=off  ShowErrorCodeOutput=on  VariableSizeOutputs=off
  Read Point Cloud : robotlib/Read Point Cloud  MaximumPointCloudSize=[ 480, 640 ]  PreserveStructure=on  ShowRGBOutput=off  ShowIntensityOutput=off  ShowErrorCodeOutput=on  VariableSizeOutputs=off
  Terminator{,1..3} (4 alike) : Terminator
  To Video Display1 : visionsinks/To Video Display  windowSizeMode=Normal  openAtMdlStart=on  fullScreen=off  videoWindowX=637  videoWindowY=276  saveWindowSize=off  videoWindowWidth=640  videoWindowHeight=480  inputColorFormat=RGB  inputType=Obsolete  imagePorts=One multidimensional signal  OutputDevice=On-screen video monitor  dataOrg=Column-major  isWindowOpen=off
  Output : Outport
  wires:
  Object Detector/1(Out1) -> Data Type Conversion/1, MATLAB System/3
  PointCloudSubscriber/2 -> Read Image/1
  ImageSubscriber/2 -> Read Point Cloud/1
  Read Image/1 -> Object Detector/1(InputImage), Draw Shapes/1, MATLAB System/2
  Read Point Cloud/1 -> MATLAB System/1
  Data Type Conversion/1 -> Draw Shapes/2
  Draw Shapes/1 -> To Video Display1/1
  Constant/1 -> Bus Assignment/1
  MATLAB System/1 -> Bus Assignment/2
  MATLAB System/2 -> Bus Assignment/3
  Bus Assignment/1 -> Output/1
  Constant1/1 -> MATLAB Function/1(objectDetectorResponseIn)
  MATLAB System/3 -> MATLAB Function/2(objectPose)
  MATLAB Function/1(objectResponseOut) -> Bus Assignment/4
  Read Image/2 -> Terminator/1
  Read Point Cloud/2 -> Terminator1/1
  ImageSubscriber/1 -> Terminator2/1
  PointCloudSubscriber/1 -> Terminator3/1

== system IntelligentBinPicking/ROSDeviceAddress Display ==

== system IntelligentBinPicking/Robot Command ==
  Input : Inport
  Bus Selector : BusSelector  OutputSignals=ProcessCommand
  Robot Command Subsystem : Subsystem  TreatAsAtomicUnit=on
  wires:
  Input/1 -> Bus Selector/1, Robot Command Subsystem/1(Input)
  Bus Selector/1 -> Robot Command Subsystem/Enable  "<ProcessCommand>"

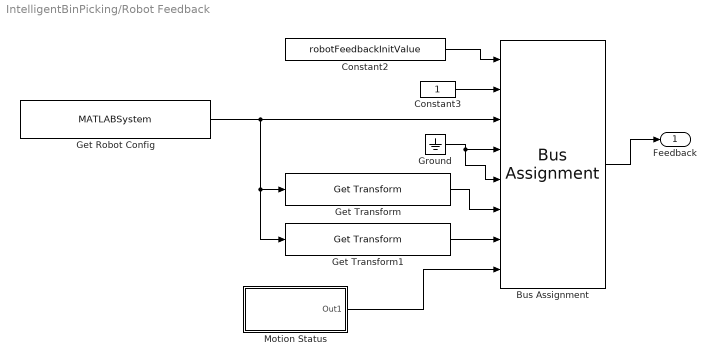
== system IntelligentBinPicking/Robot Feedback ==
  Bus Assignment : BusAssignment  AssignedSignals=IsValid,JointPos,JointVel,JointCurrent,TooltipTransform,RGBCameraTransform,IsMoving
  Constant2 : Constant  Value=robotFeedbackInitValue  OutDataTypeStr=Bus: BUS_robot_feedback
  Constant3 : Constant  OutDataTypeStr=boolean
  Get Robot Config : MATLABSystem  System=GetConfigURSO  ROSDeviceAddress=ROSDeviceAddress  SimulateUsing=Interpreted execution
      mask Type: GetConfigURSO
      mask Display:
      | disp('GetConfigURSO');
      | port_label('output',1,'config');
  Get Transform : robotmaniplib/Get Transform  RigidBodyTree=ur5e  SourceBody=tcp  TargetBody=base_link  SimulateUsing=Interpreted execution
  Get Transform1 : robotmaniplib/Get Transform  RigidBodyTree=ur5e  SourceBody=base_link  TargetBody=base_link  SimulateUsing=Interpreted execution
  Ground : Ground
  Motion Status : Subsystem  Variant=on
  Feedback : Outport  OutDataTypeStr=Bus: BUS_robot_feedback  VectorParamsAs1DForOutWhenUnconnected=off
  wires:
  Get Transform1/1 -> Bus Assignment/7
  Constant2/1 -> Bus Assignment/1
  Bus Assignment/1 -> Feedback/1
  Ground/1 -> Bus Assignment/5, Bus Assignment/4
  Get Transform/1 -> Bus Assignment/6
  Constant3/1 -> Bus Assignment/2
  Motion Status/1(Out1) -> Bus Assignment/8
  Get Robot Config/1 -> Bus Assignment/3, Get Transform1/1, Get Transform/1

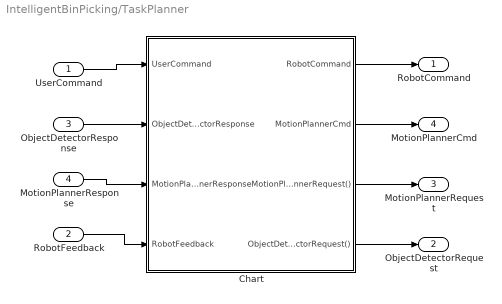
== system IntelligentBinPicking/TaskPlanner ==
  UserCommand : Inport
  RobotFeedback : Inport  Port=2  OutDataTypeStr=Bus: BUS_robot_feedback
  ObjectDetectorResponse : Inport  Port=3  OutDataTypeStr=Bus: BUS_object_detector_response
  MotionPlannerResponse : Inport  Port=4
  Chart : Stateflow chart  TreatAsAtomicUnit=on
  RobotCommand : Outport  OutDataTypeStr=Bus: BUS_robot_command  VectorParamsAs1DForOutWhenUnconnected=off
  ObjectDetectorRequest : Outport  Port=2  VectorParamsAs1DForOutWhenUnconnected=off
  MotionPlannerRequest : Outport  Port=3  VectorParamsAs1DForOutWhenUnconnected=off
  MotionPlannerCmd : Outport  Port=4  OutDataTypeStr=Bus: BUS_motion_planner_cmd  VectorParamsAs1DForOutWhenUnconnected=off
  wires:
  Chart/3(MotionPlannerRequest()) -> MotionPlannerRequest/1
  Chart/2(MotionPlannerCmd) -> MotionPlannerCmd/1
  MotionPlannerResponse/1 -> Chart/3(MotionPlannerResponse)
  Chart/4(ObjectDetectorRequest()) -> ObjectDetectorRequest/1
  ObjectDetectorResponse/1 -> Chart/2(ObjectDetectorResponse)
  Chart/1(RobotCommand) -> RobotCommand/1
  UserCommand/1 -> Chart/1(UserCommand)
  RobotFeedback/1 -> Chart/4(RobotFeedback)

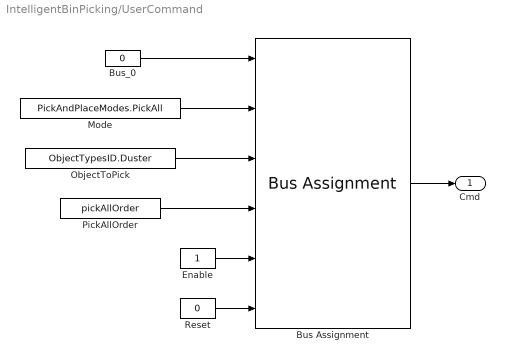
== system IntelligentBinPicking/UserCommand ==
  Bus Assignment : BusAssignment  AssignedSignals=Mode,PickSelectedObjectID,PickAllOrder,Enable,Reset
  Bus_0 : Constant  Value=0  OutDataTypeStr=Bus: BUS_user_command
  Enable : Constant  OutDataTypeStr=boolean
  Mode : Constant  Value=PickAndPlaceModes.PickAll  OutDataTypeStr=Enum: PickAndPlaceModes
  ObjectToPick : Constant  Value=ObjectTypesID.Duster
  PickAllOrder : Constant  Value=pickAllOrder
  Reset : Constant  Value=0  OutDataTypeStr=boolean
  Cmd : Outport  OutDataTypeStr=Bus: BUS_user_command  VectorParamsAs1DForOutWhenUnconnected=off
  wires:
  Bus_0/1 -> Bus Assignment/1
  Bus Assignment/1 -> Cmd/1
  ObjectToPick/1 -> Bus Assignment/3
  Enable/1 -> Bus Assignment/5
  Reset/1 -> Bus Assignment/6
  Mode/1 -> Bus Assignment/2
  PickAllOrder/1 -> Bus Assignment/4

== system IntelligentBinPicking/robotAddress Display ==

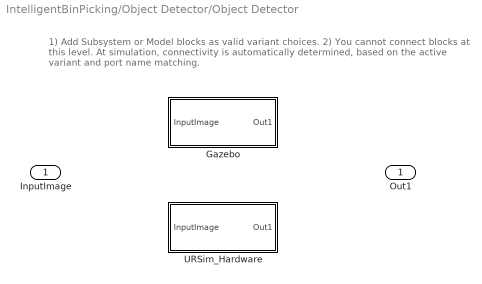
== system IntelligentBinPicking/Object Detector/Object Detector ==
  note: 1) Add Subsystem or Model blocks as valid variant choices.
      | 2) You cannot connect blocks at this level. At simulation, connectivity is automatically
      | determined, based on the active variant and port name matching.
  InputImage : Inport
  Gazebo : Subsystem  VariantControl=targetEnv == TargetEnvs.Gazebo
  URSim_Hardware : Subsystem  VariantControl=targetEnv == TargetEnvs.URSim || targetEnv == TargetEnvs.Hardware
  Out1 : Outport

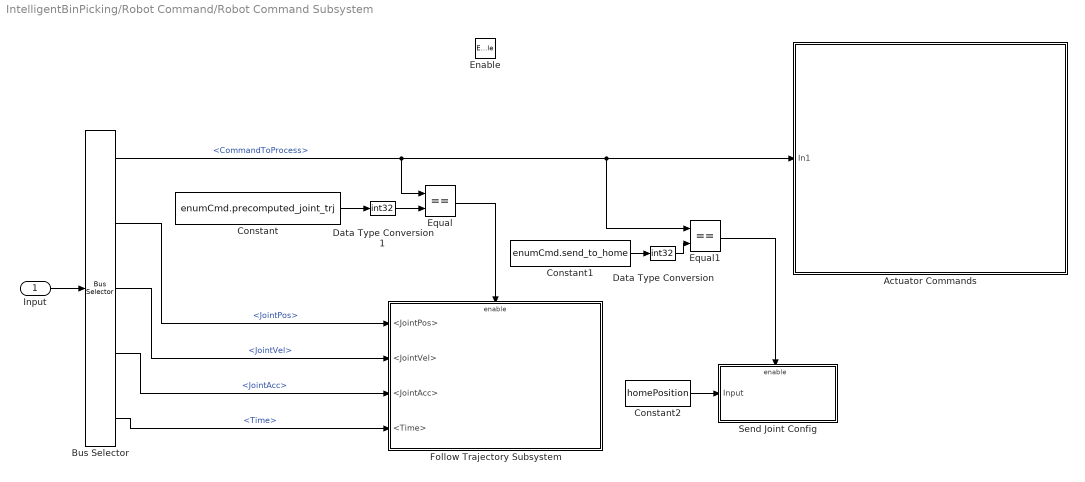
== system IntelligentBinPicking/Robot Command/Robot Command Subsystem ==
  Input : Inport
  Enable : EnablePort
  Actuator Commands : Subsystem  Variant=on
  Bus Selector : BusSelector  OutputSignals=CommandToProcess,JointTrajectory.JointPos,JointTrajectory.JointVel,JointTrajectory.JointAcc,JointTrajectory.Time
  Constant : Constant  Value=enumCmd.precomputed_joint_trj
  Constant1 : Constant  Value=enumCmd.send_to_home
  Constant2 : Constant  Value=homePosition
  Data Type Conversion : DataTypeConversion  OutDataTypeStr=int32  SaturateOnIntegerOverflow=off  RndMeth=Floor
  Data Type Conversion1 : DataTypeConversion  OutDataTypeStr=int32  SaturateOnIntegerOverflow=off  RndMeth=Floor
  Equal : RelationalOperator  Operator===  OutDataTypeStr=boolean  RndMeth=Simplest  InputSameDT=off
  Equal1 : RelationalOperator  Operator===  OutDataTypeStr=boolean  RndMeth=Simplest  InputSameDT=off
  Follow Trajectory Subsystem : Subsystem
  Send Joint Config : Subsystem  TreatAsAtomicUnit=on
  wires:
  Input/1 -> Bus Selector/1
  Bus Selector/3 -> Follow Trajectory Subsystem/2(<JointVel>)  "<JointVel>"
  Bus Selector/4 -> Follow Trajectory Subsystem/3(<JointAcc>)  "<JointAcc>"
  Bus Selector/5 -> Follow Trajectory Subsystem/4(<Time>)  "<Time>"
  Bus Selector/1 -> Actuator Commands/1(In1), Equal1/1, Equal/1  "<CommandToProcess>"
  Constant/1 -> Data Type Conversion1/1
  Equal/1 -> Follow Trajectory Subsystem/Enable
  Bus Selector/2 -> Follow Trajectory Subsystem/1(<JointPos>)  "<JointPos>"
  Constant1/1 -> Data Type Conversion/1
  Equal1/1 -> Send Joint Config/Enable
  Constant2/1 -> Send Joint Config/1(Input)
  Data Type Conversion/1 -> Equal1/2
  Data Type Conversion1/1 -> Equal/2

== system IntelligentBinPicking/Robot Feedback/Motion Status ==
  note: 1) Add Subsystem or Model blocks as valid variant choices.
      | 2) You cannot connect blocks at this level. At simulation, connectivity is automatically
      | determined, based on the active variant and port name matching.
  Gazebo : Subsystem  VariantControl=targetEnv == TargetEnvs.Gazebo
  Hardware : Subsystem  VariantControl=targetEnv == TargetEnvs.Hardware
  Out1 : Outport

== system IntelligentBinPicking/TaskPlanner/Chart/Stop ==
  f : TriggerPort  TriggerType=function-call  VariantControl=(inherit)
      settings: CopyFcn=Stateflow.SLINSF.SimulinkMan.removeBlockPreDeleteFcn  PreDeleteFcn=Stateflow.SLINSF.SimulinkMan.unsafePredeleteFcn
  Constant : Constant
  Stop Simulation : Stop
  wires:
  Constant/1 -> Stop Simulation/1

== system IntelligentBinPicking/Object Detector/Object Detector/Gazebo ==
  InputImage : Inport
  Deep Learning Object Detector : visionanalysis/Deep Learning Object Detector  Detector=Detector from MAT-file  DetectorFunction=untitled  DetectorFilePath=D:\R2023b\Simulink_BinPicking\FF\intelligent-bin-picking-simulink-example-main\Perception\trainedYOLOv4DetectorSimGazebo_cuboid.mat  MaxDetections=8  Bboxes=on  Scores=off  UseROI=off  ROI=[1 1 100 100]  Threshold=0.5  NumStrongestRegions=2000  UseMinSize=off  MinSize=[1 1]  UseMaxSize=off  MaxSize=[50 50]  ForceInterpretedSim=off
  Out1 : Outport
  wires:
  InputImage/1 -> Deep Learning Object Detector/1
  Deep Learning Object Detector/1 -> Out1/1

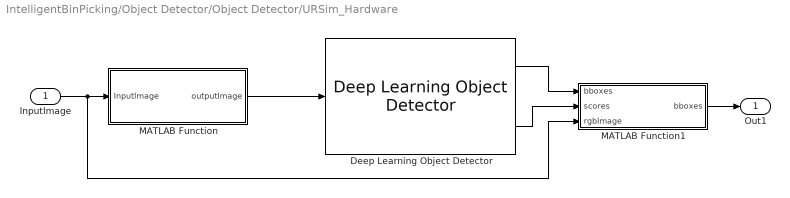
== system IntelligentBinPicking/Object Detector/Object Detector/URSim_Hardware ==
  InputImage : Inport
  Deep Learning Object Detector : visionanalysis/Deep Learning Object Detector  Detector=Detector from MAT-file  DetectorFunction=untitled  DetectorFilePath=D:\R2023a\intelligent-semi-structured-bin-picking-with-ur5e-hardware-and-intelrealsense-main\intelligent-semi-structured-bin-picking-with-ur5e-hardware-and-intelrealsense-main\MATLAB Project\Perception\trainedYOLOv4Detector_cuboid.mat  MaxDetections=15  Bboxes=on  Scores=on  UseROI=off  ROI=[1 1 100 100]  Threshold=0.5  NumStrongestRegions=2000  UseMinSize=off  MinSize=[1 1]  UseMaxSize=off  MaxSize=[50 50]  ForceInterpretedSim=off
  MATLAB Function : MATLAB Function  TreatAsAtomicUnit=on
  MATLAB Function1 : MATLAB Function  TreatAsAtomicUnit=on
  Out1 : Outport
  wires:
  InputImage/1 -> MATLAB Function1/3(rgbImage), MATLAB Function/1(InputImage)
  MATLAB Function/1(outputImage) -> Deep Learning Object Detector/1
  Deep Learning Object Detector/1 -> MATLAB Function1/1("bboxes ")
  MATLAB Function1/1(bboxes) -> Out1/1
  Deep Learning Object Detector/2 -> MATLAB Function1/2(scores)

== system IntelligentBinPicking/Robot Command/Robot Command Subsystem/Actuator Commands ==
  In1 : Inport
  Gazebo : Subsystem  VariantControl=targetEnv == TargetEnvs.Gazebo
  Hardware : Subsystem  VariantControl=targetEnv == TargetEnvs.Hardware

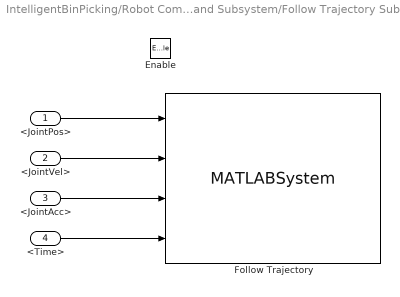
== system IntelligentBinPicking/Robot Command/Robot Command Subsystem/Follow Trajectory Subsystem ==
  <JointPos> : Inport
  <JointVel> : Inport  Port=2
  <JointAcc> : Inport  Port=3
  <Time> : Inport  Port=4
  Enable : EnablePort
  Follow Trajectory : MATLABSystem  System=FollowTrajectorySO  ROSDeviceAddress=ROSDeviceAddress  SimulateUsing=Interpreted execution
      mask Type: FollowTrajectorySO
      mask Display:
      | disp('FollowTrajectorySO');
      | port_label('input',1,'q_interp');
      | port_label('input',2,'qd_interp');
      | port_label('input',3,'qdd_interp');
      | port_label('input',4,'tSample');
  wires:
  <JointVel>/1 -> Follow Trajectory/2
  <JointAcc>/1 -> Follow Trajectory/3
  <JointPos>/1 -> Follow Trajectory/1
  <Time>/1 -> Follow Trajectory/4

== system IntelligentBinPicking/Robot Command/Robot Command Subsystem/Send Joint Config ==
  Input : Inport
  Enable : EnablePort
  MATLAB System : MATLABSystem  System=SendJointConfigSO  ROSDeviceAddress=ROSDeviceAddress  SimulateUsing=Interpreted execution
      mask Type: SendJointConfigSO
      mask Display:
      | disp('SendJointConfigSO');
      | port_label('input',1,'config');
  wires:
  Input/1 -> MATLAB System/1

== system IntelligentBinPicking/Robot Feedback/Motion Status/Gazebo ==
  Constant : Constant  Value=false
  Out1 : Outport
  wires:
  Constant/1 -> Out1/1

== system IntelligentBinPicking/Robot Feedback/Motion Status/Hardware ==
  MATLAB System : MATLABSystem  System=MotionStatusUR  ROSDeviceAddress=ROSDeviceAddress
      mask Type: MotionStatusUR
      mask Display:
      | disp('MotionStatusUR');
      | port_label('output',1,'success');
  NOT : Logic  Operator=NOT  AllPortsSameDT=off  OutDataTypeStr=boolean
  Out1 : Outport
  wires:
  MATLAB System/1 -> NOT/1
  NOT/1 -> Out1/1

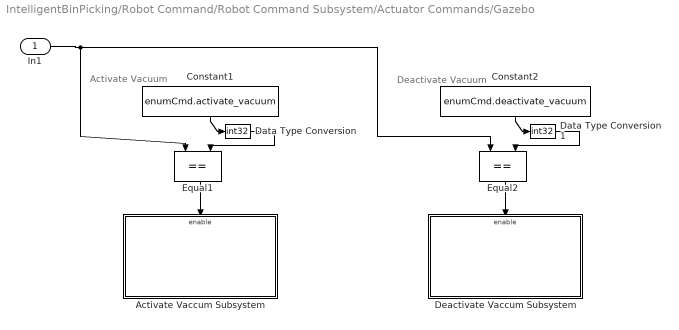
== system IntelligentBinPicking/Robot Command/Robot Command Subsystem/Actuator Commands/Gazebo ==
  note: Deactivate Vacuum
  note: Activate Vacuum
  In1 : Inport
  Activate Vaccum Subsystem : Subsystem
  Constant1 : Constant  Value=enumCmd.activate_vacuum
  Constant2 : Constant  Value=enumCmd.deactivate_vacuum
  Data Type Conversion : DataTypeConversion  OutDataTypeStr=int32  SaturateOnIntegerOverflow=off  RndMeth=Floor
  Data Type Conversion1 : DataTypeConversion  OutDataTypeStr=int32  SaturateOnIntegerOverflow=off  RndMeth=Floor
  Deactivate Vaccum Subsystem : Subsystem
  Equal1 : RelationalOperator  Operator===  OutDataTypeStr=boolean  RndMeth=Simplest  InputSameDT=off
  Equal2 : RelationalOperator  Operator===  OutDataTypeStr=boolean  RndMeth=Simplest  InputSameDT=off
  wires:
  Constant1/1 -> Data Type Conversion/1
  Equal2/1 -> Deactivate Vaccum Subsystem/Enable
  Constant2/1 -> Data Type Conversion1/1
  Equal1/1 -> Activate Vaccum Subsystem/Enable
  In1/1 -> Equal2/1, Equal1/1
  Data Type Conversion/1 -> Equal1/2
  Data Type Conversion1/1 -> Equal2/2

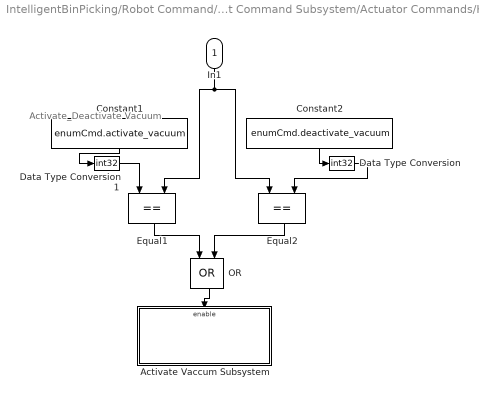
== system IntelligentBinPicking/Robot Command/Robot Command Subsystem/Actuator Commands/Hardware ==
  note: Activate_Deactivate Vacuum
  In1 : Inport
  Activate Vaccum Subsystem : Subsystem
  Constant1 : Constant  Value=enumCmd.activate_vacuum
  Constant2 : Constant  Value=enumCmd.deactivate_vacuum
  Data Type Conversion : DataTypeConversion  OutDataTypeStr=int32  SaturateOnIntegerOverflow=off  RndMeth=Floor
  Data Type Conversion1 : DataTypeConversion  OutDataTypeStr=int32  SaturateOnIntegerOverflow=off  RndMeth=Floor
  Equal1 : RelationalOperator  Operator===  OutDataTypeStr=boolean  RndMeth=Simplest  InputSameDT=off
  Equal2 : RelationalOperator  Operator===  OutDataTypeStr=boolean  RndMeth=Simplest  InputSameDT=off
  OR : Logic  Operator=OR  AllPortsSameDT=off  OutDataTypeStr=boolean
  wires:
  Constant1/1 -> Data Type Conversion1/1
  Equal1/1 -> OR/1
  In1/1 -> Equal1/2, Equal2/1
  Constant2/1 -> Data Type Conversion/1
  Equal2/1 -> OR/2
  OR/1 -> Activate Vaccum Subsystem/Enable
  Data Type Conversion/1 -> Equal2/2
  Data Type Conversion1/1 -> Equal1/1

== system IntelligentBinPicking/Robot Command/Robot Command Subsystem/Actuator Commands/Gazebo/Activate Vaccum Subsystem ==
  Enable : EnablePort
  Activate Vacuum : robotlib/Call Service  topicSource=Select from ROS network  service=/ur5/epick1/on  serviceType=std_srvs/Empty  connectionTimeout=5  keepPersistent=off  ShowErrorCodeOutput=on  legacyBusStruct=off
  Blank Message : robotlib/Blank Message  messageClass=Service Request  entityType=std_srvs/Empty  messageType=std_srvs/EmptyRequest  SampleTime=inf  legacyBusStruct=off
  wires:
  Blank Message/1 -> Activate Vacuum/1

== system IntelligentBinPicking/Robot Command/Robot Command Subsystem/Actuator Commands/Gazebo/Deactivate Vaccum Subsystem ==
  Enable : EnablePort
  Blank Message : robotlib/Blank Message  messageClass=Service Request  entityType=std_srvs/Empty  messageType=std_srvs/EmptyRequest  SampleTime=inf  legacyBusStruct=off
  Deactivate Vacuum : robotlib/Call Service  topicSource=Select from ROS network  service=/ur5/epick1/off  serviceType=std_srvs/Empty  connectionTimeout=5  keepPersistent=off  ShowErrorCodeOutput=on  legacyBusStruct=off
  wires:
  Blank Message/1 -> Deactivate Vacuum/1
